simulink model "project1"  (R2017a)
settings: Solver=VariableStepAuto  StartTime=0.0  StopTime=10.0  RelTol=1e-3
libraries: simulink x8
settings Model: Creator=Administrator  LastModifiedBy=Administrator

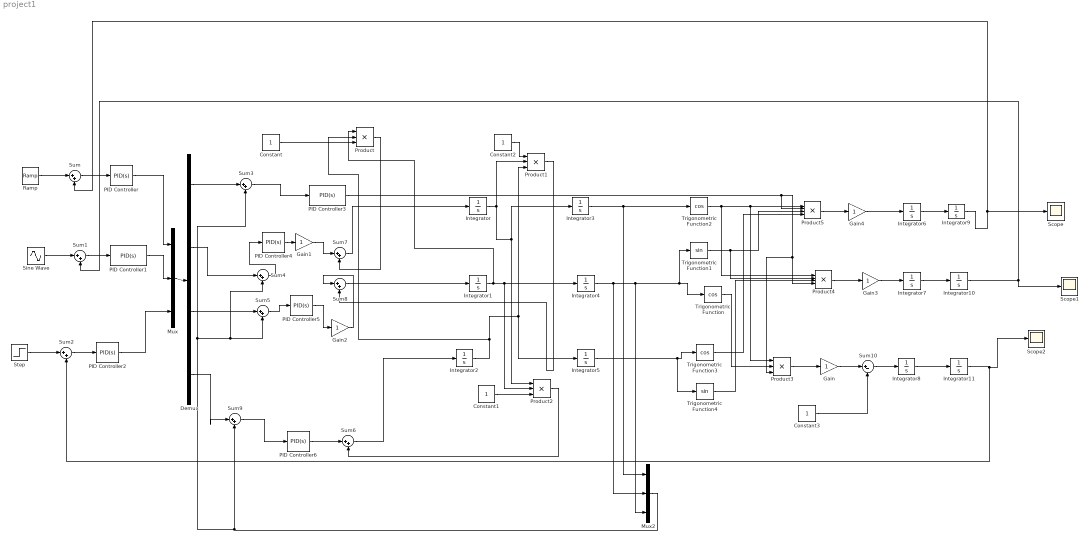
== system project1 ==
  Constant{,1..3} (4 alike) : Constant
  Demux : Demux
  Gain{,1..4} (5 alike) : Gain
  Integrator{,1..11} (12 alike) : Integrator
  Mux : Mux  Inputs=3
  Mux2 : Mux  Inputs=3
  PID Controller{,1..6} (7 alike) : simulink/Continuous/PID Controller  Controller=PID  TimeDomain=Continuous-time  SampleTime=-1  IntegratorMethod=Forward Euler  FilterMethod=Forward Euler  Form=Parallel  UseFilter=on  ControllerParametersSource=internal  P=1  I=1  D=0  N=100  InitialConditionSource=internal  InitialConditionForIntegrator=0  InitialConditionForFilter=0  ExternalReset=none  LimitOutput=off  UpperSaturationLimit=inf  LowerSaturationLimit=-inf  LinearizeAsGain=on  AntiWindupMode=none  Kb=1  TrackingMode=off  Kt=1  PParamMin=[]  PParamMax=[]  IParamMin=[]  IParamMax=[]  DParamMin=[]  DParamMax=[]  NParamMin=[]  NParamMax=[]  KbParamMin=[]  KbParamMax=[]  KtParamMin=[]  KtParamMax=[]  POutMin=[]  POutMax=[]  IOutMin=[]  IOutMax=[]  DOutMin=[]  DOutMax=[]  NOutMin=[]  NOutMax=[]  KbOutMin=[]  KbOutMax=[]  KtOutMin=[]  KtOutMax=[]  IntegratorOutMin=[]  IntegratorOutMax=[]  FilterOutMin=[]  FilterOutMax=[]  SumOutMin=[]  SumOutMax=[]  SumI1OutMin=[]  SumI1OutMax=[]  SumI2OutMin=[]  SumI2OutMax=[]  SumI3OutMin=[]  SumI3OutMax=[]  SumDOutMin=[]  SumDOutMax=[]  SaturationOutMin=[]  SaturationOutMax=[]  IntegratorContinuousStateAttributes=''  IntegratorStateMustResolveToSignalObject=off  IntegratorRTWStateStorageClass=Auto  FilterContinuousStateAttributes=''  FilterStateMustResolveToSignalObject=off  FilterRTWStateStorageClass=Auto  DifferentiatorICPrevScaledInput=0  DifferentiatorOutMin=[]  DifferentiatorOutMax=[]  InitialConditionSetting=State (most efficient)
  Product{,1..3} (4 alike) : Product  Inputs=3
  Product4 : Product  Inputs=4
  Product5 : Product  Inputs=4
  Ramp : simulink/Sources/Ramp  slope=1  start=0  X0=0
  Scope : Scope
  Scope1 : Scope
  Scope2 : Scope
  Sine Wave : Sin  SampleTime=0
  Step : Step  SampleTime=0
  Sum{,1..9} (10 alike) : Sum  Inputs=|++
  Sum10 : Sum  Inputs=|+-
  Trigonometric Function : Trigonometry  Operator=cos
  Trigonometric Function1 : Trigonometry
  Trigonometric Function2 : Trigonometry  Operator=cos
  Trigonometric Function3 : Trigonometry  Operator=cos
  Trigonometric Function4 : Trigonometry
  wires:
  Sum/1 -> PID Controller/1
  Ramp/1 -> Sum/1
  Sine Wave/1 -> Sum1/1
  Sum1/1 -> PID Controller1/1
  Step/1 -> Sum2/1
  Sum2/1 -> PID Controller2/1
  PID Controller/1 -> Mux/1
  PID Controller1/1 -> Mux/2
  PID Controller2/1 -> Mux/3
  Mux/1 -> Demux/1
  Demux/1 -> Sum3/1
  Sum3/1 -> PID Controller3/1
  Demux/2 -> Sum4/1
  Sum4/1 -> PID Controller4/1
  Demux/3 -> Sum5/1
  Sum5/1 -> PID Controller5/1
  PID Controller4/1 -> Gain1/1
  PID Controller5/1 -> Gain2/1
  Gain1/1 -> Sum7/1
  Gain2/1 -> Sum8/1
  Integrator/1 -> Product2/1, Integrator3/1, Product1/2
  Integrator2/1 -> Product1/3, Integrator5/1, Product/2
  Integrator1/1 -> Product/1, Product2/2, Integrator4/1
  Constant/1 -> Product/3
  Constant1/1 -> Product2/3
  Constant2/1 -> Product1/1
  Integrator4/1 -> Mux2/2, Mux2/3, Trigonometric Function1/1, Trigonometric Function/1
  Integrator3/1 -> Mux2/1, Trigonometric Function2/1
  Integrator5/1 -> Trigonometric Function4/1, Trigonometric Function3/1
  Trigonometric Function2/1 -> Product4/1, Product3/1, Product5/1
  Trigonometric Function1/1 -> Product4/2, Product5/3
  Trigonometric Function3/1 -> Product5/4
  Trigonometric Function4/1 -> Product4/3
  Trigonometric Function/1 -> Product3/2
  Demux/4 -> Sum9/1
  Sum9/1 -> PID Controller6/1
  Product/1 -> Sum7/2
  Product1/1 -> Sum8/2
  PID Controller6/1 -> Sum6/1
  Product2/1 -> Sum6/2
  Sum7/1 -> Integrator/1
  Sum8/1 -> Integrator1/1
  Sum6/1 -> Integrator2/1
  PID Controller3/1 -> Product3/3, Product4/4, Product5/2
  Constant3/1 -> Sum10/2
  Product5/1 -> Gain4/1
  Product4/1 -> Gain3/1
  Product3/1 -> Gain/1
  Gain/1 -> Sum10/1
  Sum10/1 -> Integrator8/1
  Gain3/1 -> Integrator7/1
  Gain4/1 -> Integrator6/1
  Integrator6/1 -> Integrator9/1
  Integrator7/1 -> Integrator10/1
  Integrator8/1 -> Integrator11/1
  Mux2/1 -> Sum5/2, Sum4/2, Sum3/2, Sum9/2
  Integrator9/1 -> Scope/1, Sum/2
  Integrator10/1 -> Scope1/1, Sum1/2
  Integrator11/1 -> Scope2/1, Sum2/2
